simulink model "RigidBody6dof2016a"  (R2016a)
settings: Solver=ode45  SolverMode=SingleTasking  StartTime=0.0  StopTime=10.0  RelTol=1e-3
libraries: simulink_extras x3
settings Model: Creator=andrealunaro  LastModifiedBy=andrealunaro
settings DataIOCC: ReturnWorkspaceOutputs=on
settings DebuggingCC: SFUnexpectedBacktrackingDiag=error  SFNoUnconditionalDefaultTransitionDiag=error
settings HardwareCC: ProdWordSize=32  ProdHWDeviceType=Specified
settings SFSimCC: SimUseLocalCustomCode=on
settings RTWCC: RTWUseLocalCustomCode=on
settings GRTTargetCC: TargetLangStandard=C99 (ISO)
settings ConfigComp: CovMetricSettings=dwe  CovSaveCumulativeToWorkspaceVar=off  CovSaveSingleToWorkspaceVar=off  CovExternalEMLEnable=on

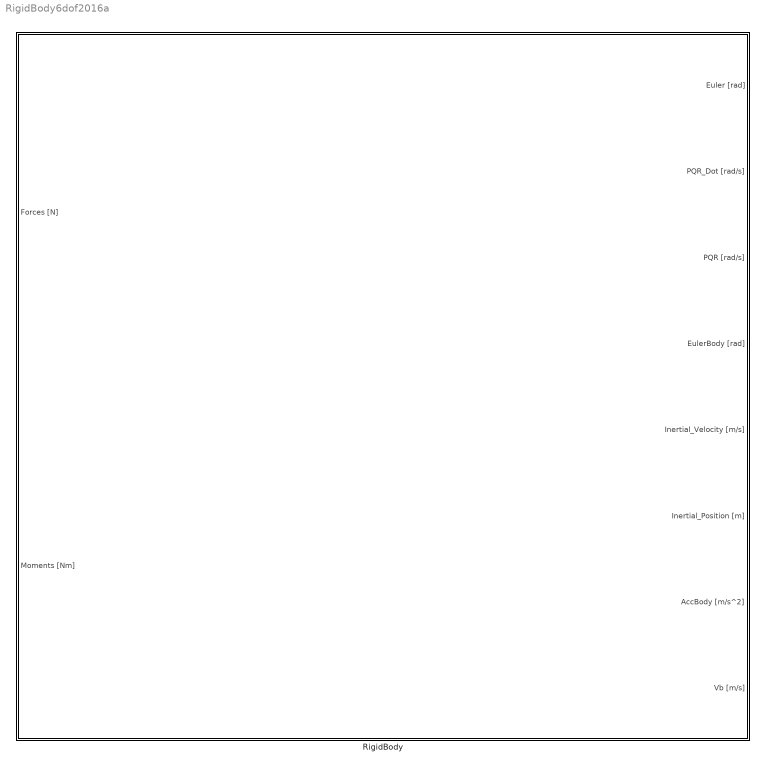
== system RigidBody6dof2016a ==
  RigidBody : Subsystem  mask{Phi_init=0, Theta_init=0, Psi_init=0, Inertial_Position_init=[0;0;0], P_init=0, Q_init=0, R_init=0, Ub_init=0, Vb_init=0, Wb_init=0, phiB_init=0, thetaB_init=0, psiB_init=0, RigidBodyInertia=0, RigidBodyMass=0}
      mask prompts: RigidBodyInertia "Rigid Body Inertia [kg m^2]"; RigidBodyMass "Rigid Body Mass [kg]"
      mask DialogControl DescGroupVar Prompt: 6DOF rigid body model
      mask DialogControl DescTextVar Prompt: Integrate the six-degrees-of-freedom equations of motion in body axis.
      mask DialogControl Container16 Prompt: Rigid Body Parameters
      mask Display: image('x6DofRB1.png')

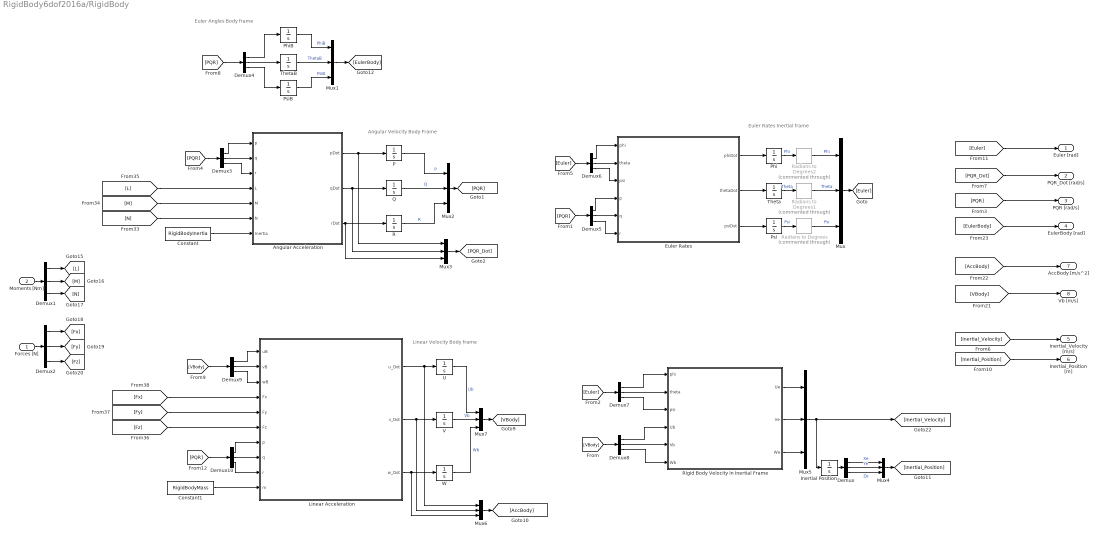
== system RigidBody6dof2016a/RigidBody ==
  note: Euler Rates Inertial frame
  note: Angular Velocity Body Frame
  note: Linear Velocity Body frame
  note: Euler Angles Body frame
  Forces [N] : Inport
  Moments [Nm] : Inport  Port=2
  Angular Acceleration : MATLAB Function  TreatAsAtomicUnit=on
  Constant : Constant  Value=RigidBodyInertia
  Constant1 : Constant  Value=RigidBodyMass
  Demux{,1..10} (11 alike) : Demux  Outputs=3
  Euler Rates : MATLAB Function  TreatAsAtomicUnit=on
  Inertial Position : Integrator  InitialCondition=Inertial_Position_init  ContinuousStateAttributes={'xe', 'ye', 'ze'}
  Linear Acceleration : MATLAB Function  TreatAsAtomicUnit=on
  Mux{,1..7} (8 alike) : Mux  Inputs=3
  P : Integrator  InitialCondition=P_init  UpperSaturationLimit=5  LowerSaturationLimit=-5  ContinuousStateAttributes='P'
  Phi : Integrator  InitialCondition=Phi_init  UpperSaturationLimit=pi/6  LowerSaturationLimit=-pi/6  WrapState=on  ContinuousStateAttributes='Phi'
  PhiB : Integrator  InitialCondition=phiB_init  WrapState=on  ContinuousStateAttributes='PhiB'
  Psi : Integrator  InitialCondition=Psi_init  UpperSaturationLimit=pi  LowerSaturationLimit=-pi  WrapState=on  ContinuousStateAttributes='Psi'
  PsiB : Integrator  InitialCondition=psiB_init  WrapState=on  ContinuousStateAttributes='PsiB'
  Q : Integrator  InitialCondition=Q_init  UpperSaturationLimit=5  LowerSaturationLimit=-5  ContinuousStateAttributes='Q'
  R : Integrator  InitialCondition=R_init  UpperSaturationLimit=5  LowerSaturationLimit=-5  ContinuousStateAttributes='R'
  Radians to Degrees : simulink_extras/Transformations/Radians to Degrees  Commented=through
  Radians to Degrees1 : simulink_extras/Transformations/Radians to Degrees  Commented=through
  Radians to Degrees2 : simulink_extras/Transformations/Radians to Degrees  Commented=through
  "Rigid Body Velocity in Inertial Frame " : MATLAB Function  TreatAsAtomicUnit=on
  Theta : Integrator  InitialCondition=Theta_init  UpperSaturationLimit=pi/6  LowerSaturationLimit=-pi/6  WrapState=on  ContinuousStateAttributes='Theta'
  ThetaB : Integrator  InitialCondition=thetaB_init  WrapState=on  ContinuousStateAttributes='ThetaB'
  U : Integrator  InitialCondition=Ub_init  UpperSaturationLimit=100  LowerSaturationLimit=-30  ContinuousStateAttributes='uB'
  V : Integrator  InitialCondition=Vb_init  UpperSaturationLimit=5  LowerSaturationLimit=-5  ContinuousStateAttributes='vB'
  W : Integrator  InitialCondition=Wb_init  UpperSaturationLimit=3  LowerSaturationLimit=-10  ContinuousStateAttributes='wB'
  Euler [rad] : Outport
  PQR_Dot [rad/s] : Outport  Port=2
  PQR [rad/s] : Outport  Port=3
  "EulerBody [rad] " : Outport  Port=4
  Inertial_Velocity [m/s] : Outport  Port=5
  "Inertial_Position [m] " : Outport  Port=6
  AccBody [m/s^2] : Outport  Port=7
  Vb [m/s] : Outport  Port=8
  wires:
  Demux6/1 -> Euler Rates/1(phi)
  [Euler] -> Euler [rad]/1
  Demux6/2 -> Euler Rates/2(theta)
  Demux6/3 -> Euler Rates/3(psi)
  Linear Acceleration/1(u_Dot) -> Mux6/1, U/1
  Linear Acceleration/2(v_Dot) -> Mux6/2, V/1
  [PQR] -> PQR [rad/s]/1
  Demux3/1 -> Angular Acceleration/1(p)
  Demux3/2 -> Angular Acceleration/2(q)
  Demux3/3 -> Angular Acceleration/3(r)
  Demux9/3 -> Linear Acceleration/3(wB)
  Demux9/2 -> Linear Acceleration/2(vB)
  V/1 -> Mux7/2  "Vb"
  W/1 -> Mux7/3  "Wb"
  Demux8/1 -> "Rigid Body Velocity in Inertial Frame "/4(Ub)
  Demux8/3 -> "Rigid Body Velocity in Inertial Frame "/6(Wb)
  Demux8/2 -> "Rigid Body Velocity in Inertial Frame "/5(Vb)
  "Rigid Body Velocity in Inertial Frame "/3(We) -> Mux5/3
  "Rigid Body Velocity in Inertial Frame "/2(Ve) -> Mux5/2
  Mux5/1 -> Inertial Position/1, [Inertial_Velocity]
  "Rigid Body Velocity in Inertial Frame "/1(Ue) -> Mux5/1
  [Inertial_Velocity] -> Inertial_Velocity [m/s]/1
  [Inertial_Position] -> "Inertial_Position [m] "/1
  Demux/1 -> Mux4/1  "Xe"
  Demux/2 -> Mux4/2  "Ye"
  Mux4/1 -> [Inertial_Position]
  Constant/1 -> Angular Acceleration/7(Inertia)
  Constant1/1 -> Linear Acceleration/10(m)
  [Fy] -> Linear Acceleration/5(Fy)
  Linear Acceleration/3(w_Dot) -> Mux6/3, W/1
  [Fz] -> Linear Acceleration/6(Fz)
  [Fx] -> Linear Acceleration/4(Fx)
  [M] -> Angular Acceleration/5(M)
  [L] -> Angular Acceleration/4(L)
  [N] -> Angular Acceleration/6(N)
  [AccBody] -> AccBody [m/s^2]/1
  [PQR_Dot] -> PQR_Dot [rad/s]/1
  [EulerBody] -> "EulerBody [rad] "/1
  PhiB/1 -> Mux1/1  "PhiB"
  ThetaB/1 -> Mux1/2  "ThetaB"
  PsiB/1 -> Mux1/3  "PsiB"
  P/1 -> Mux2/1  "P"
  Angular Acceleration/3(rDot) -> Mux3/3, R/1
  Q/1 -> Mux2/2  "Q"
  Angular Acceleration/2(qDot) -> Mux3/2, Q/1
  Angular Acceleration/1(pDot) -> Mux3/1, P/1
  Euler Rates/1(phiDot) -> Phi/1
  Radians to Degrees/1 -> Mux/3  "Psi"
  Radians to Degrees1/1 -> Mux/2  "Theta"
  Psi/1 -> Radians to Degrees/1  "Psi"
  Euler Rates/3(psiDot) -> Psi/1
  Radians to Degrees2/1 -> Mux/1  "Phi"
  Theta/1 -> Radians to Degrees1/1  "Theta"
  Euler Rates/2(thetaDot) -> Theta/1
  Phi/1 -> Radians to Degrees2/1  "Phi"
  U/1 -> Mux7/1  "Ub"
  Demux/3 -> Mux4/3  "Ze"
  Inertial Position/1 -> Demux/1
  Moments [Nm]/1 -> Demux1/1
  Demux1/1 -> [L]
  Demux1/2 -> [M]
  Demux1/3 -> [N]
  Demux2/3 -> [Fz]
  Demux2/2 -> [Fy]
  Demux2/1 -> [Fx]
  Mux7/1 -> [VBody]
  [VBody] -> Vb [m/s]/1
  Mux6/1 -> [AccBody]
  Mux1/1 -> [EulerBody]
  R/1 -> Mux2/3  "R"
  Mux2/1 -> [PQR]
  Mux3/1 -> [PQR_Dot]
  Mux/1 -> [Euler]
  [PQR] -> Demux3/1
  Demux4/1 -> PhiB/1
  Demux4/2 -> ThetaB/1
  Demux4/3 -> PsiB/1
  [PQR] -> Demux4/1
  [VBody] -> Demux9/1
  Demux9/1 -> Linear Acceleration/1(uB)
  Demux10/1 -> Linear Acceleration/7(p)
  Demux10/2 -> Linear Acceleration/8(q)
  Demux10/3 -> Linear Acceleration/9(r)
  [PQR] -> Demux10/1
  [Euler] -> Demux6/1
  Demux5/1 -> Euler Rates/4(p)
  [PQR] -> Demux5/1
  Demux7/1 -> "Rigid Body Velocity in Inertial Frame "/1(phi)
  Demux7/2 -> "Rigid Body Velocity in Inertial Frame "/2(theta)
  Demux7/3 -> "Rigid Body Velocity in Inertial Frame "/3(psi)
  [Euler] -> Demux7/1
  [VBody] -> Demux8/1
  Forces [N]/1 -> Demux2/1
  Demux5/2 -> Euler Rates/5(q)
  Demux5/3 -> Euler Rates/6(r)

== matlab function RigidBody6dof2016a/RigidBody/Linear Acceleration ==
  data: uB input; vB input; wB input; Fx input; u_Dot output; Fy input; Fz input; p input; q input; r input; v_Dot output; w_Dot output; m input
function [u_Dot, v_Dot, w_Dot] = AccLin(uB, vB, wB, Fx, Fy, Fz, p, q, r, m)



Fb = [Fx; Fy; Fz];
omega = [p; q; r];
Vb = [uB; vB; wB];

Accelerations = (1/m*Fb - cross(omega,Vb));

% u_Dot = Fx/m + vB*r - wB*q;
% v_Dot = Fy/m - uB*r + wB*p;
% w_Dot = Fz/m + uB*q - vB*p;


u_Dot = Accelerations(1);
v_Dot = Accelerations(2);
w_Dot = Accelerations(3);
end

== matlab function RigidBody6dof2016a/RigidBody/Angular Acceleration ==
  data: p input; pDot output; q input; r input; L input; M input; N input; qDot output; rDot output; Inertia input
function [pDot,qDot, rDot] = AccAng(p, q, r, L, M , N, Inertia)




% Ixx      = 146.68;  
% Iyy      = 457.67;
% Izz      = 440.70;

Ixx      = Inertia(1,1); 
Ixy      = Inertia(1,2); 
Ixz      = Inertia(1,3); 


Iyx      = Inertia(2,1);
Iyy      = Inertia(2,2);
Iyz      = Inertia(2,3);


Izx      = Inertia(3,1);
Izy      = Inertia(3,2);
Izz      = Inertia(3,3);

I        =  [Ixx, Ixy, Ixz;
             Iyx, Iyy, Iyz;
             Izx, Izy, Izz];
         
omega    = [p; q; r];         
Moments  = [L; M; N];
Iomega   = I*omega;

omegaDot = I^-1*(Moments - cross(omega,Iomega)); 
 
% pDot     = ((Iyy - Izz)*q*r+L)/Ixx;
% qDot     = ((-Ixx + Izz)*p*r+M)/Iyy;
% rDot     = ((Ixx - Iyy)*p*q+N)/Izz;

pDot     = omegaDot(1);
qDot     = omegaDot(2);
rDot     = omegaDot(3);

end

== matlab function RigidBody6dof2016a/RigidBody/Euler Rates ==
  data: phi input; phiDot output; theta input; psi input; p input; q input; r input; thetaDot output; psiDot output
function [phiDot, thetaDot, psiDot] = VangS2B(phi, theta, psi, p, q, r)

phi      = deg2rad(phi);
theta    = deg2rad(theta);
psi      = deg2rad(psi);


phiDot   = p+sin(phi)*tan(theta)*q+cos(phi)*tan(theta)*r;

thetaDot = cos(phi)*q-sin(phi)*r;

psiDot   = sin(phi)/cos(theta)*q+cos(phi)/cos(theta)*r;

end

== matlab function RigidBody6dof2016a/RigidBody/Rigid Body Velocity in Inertial Frame  ==
  data: phi input; theta input; psi input; Ub input; Vb input; Wb input; Ue output; Ve output; We output
function [Ue, Ve, We] = RotS2B(phi,theta, psi, Ub, Vb, Wb)

phi      = deg2rad(phi);
theta    = deg2rad(theta);
psi      = deg2rad(psi);

R = [ cos(theta)*cos(psi), cos(theta)*sin(psi), -sin(theta);
    sin(phi)*sin(theta)*cos(psi)-cos(phi)*sin(psi), sin(phi)*sin(theta)*sin(psi)+cos(phi)*cos(psi), sin(phi)*cos(theta);
    cos(phi)*sin(theta)*cos(psi)+sin(phi)*sin(psi), cos(phi)*sin(theta)*sin(psi)-sin(phi)*cos(psi), cos(phi)*cos(theta)];
    

p = [Ub; Vb; Wb];
p = R'*p; 

Ue = p(1);
Ve = p(2);
We = p(3);

end
